simulink model "RC_Circuit"  (R2024a)
settings: Solver=FixedStepDiscrete  StartTime=0.0  StopTime=10.0  FixedStep=1E-3  RelTol=1e-3
values from neighbouring files (symbols this model uses):
  C = 1E-6    (= 1e-06)    [RC.m]
  R = 1000    [RC.m]
settings Model: Creator=VICTUS  LastModifiedBy=VICTUS

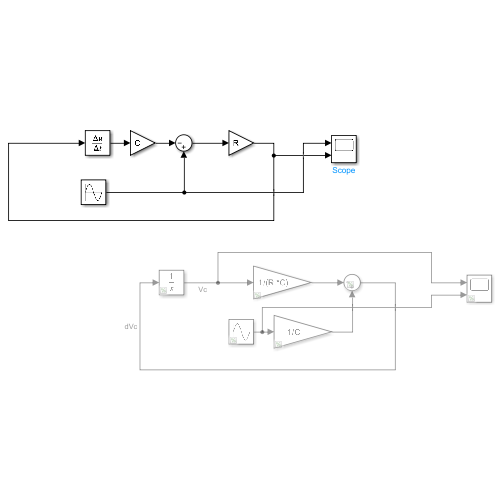
[thumbnail: Simulink's stored preview of the top-level diagram]
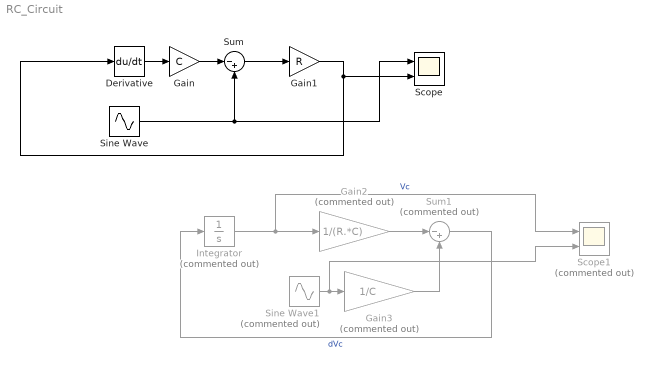
== system RC_Circuit ==
  Derivative : Derivative
  Gain : Gain  Gain=C
  Gain1 : Gain  Gain=R
  Gain2 : Gain  Commented=on  Gain=1/(R.*C)
  Gain3 : Gain  Commented=on  Gain=1/C
  Integrator : Integrator  Commented=on
  Scope : Scope  NumInputPorts=2
  Scope1 : Scope  Commented=on  NumInputPorts=2
  Sine Wave : Sin  Amplitude=5  Frequency=2*pi  SampleTime=0
  Sine Wave1 : Sin  Commented=on  Amplitude=5  Frequency=2*pi  SampleTime=0
  Sum : Sum  Inputs=|-+
  Sum1 : Sum  Commented=on  Inputs=|-+
  wires:
  Gain1/1 -> Derivative/1, Scope/2
  Derivative/1 -> Gain/1
  Gain/1 -> Sum/1
  Sine Wave/1 -> Sum/2, Scope/1
  Sum/1 -> Gain1/1
  Integrator/1 -> Scope1/1, Gain2/1  "Vc"
  Sum1/1 -> Integrator/1  "dVc"
  Gain2/1 -> Sum1/1
  Sine Wave1/1 -> Scope1/2, Gain3/1
  Gain3/1 -> Sum1/2
